simulink model "ECUDamperRR"  (Simulink 7.7)
settings: Solver=ode3  StartTime=0.0  StopTime=10.0  FixedStep=T  RelTol=1e-3
values from neighbouring files (symbols this model uses):
  Suspension =     [VehicleData_VectorCar.mat]
libraries: canoelib x5
settings Model: Creator=vishc  LastModifiedBy=visjf
settings DataIOCC: SaveOutput=off  SignalLogging=off  SaveTime=off
settings OptimizationCC: InlineParams=on  UseIntDivNetSlope=on
settings DebuggingCC: StrictBusMsg=Warning
settings SFSimCC: SimParseCustomCode=off
settings RTWCC: SystemTargetFile=cn.tlc  TemplateMakefile=cn_msdll.tmf  Description=Vector CANoe Real-Time Target DLL (Visual C/C++ Project Makefile)  ProcessScript=cn_make_rtw_hook
settings CodeAppCC: MaxIdLength=128  SimulinkBlockComments=off
settings STFCustomTargetCC: FunctionExecutionProfile=off  GeneratePreprocessorConditionals=Disable all  MatFileLogging=on  SystemTargetFile=cn.tlc
settings GRTTargetCC: ParMdlRefBuildCompliant=off  CompOptLevelCompliant=off  ExtModeMexFile=noextcomm  RTWCAPISignals=on  RTWCAPIParams=on
settings CustomProperty: DataType=string  Value=..\canoe

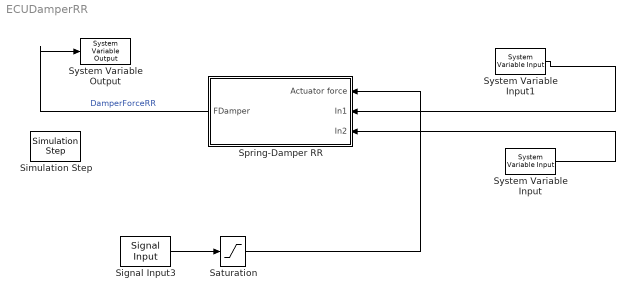
== system ECUDamperRR ==
  Saturation : Saturate  UpperLimit=6e3  LowerLimit=-6e3
  Signal Input3 : canoelib/CANoe I//O/Signal Input  SystemSampleTime=-1  dbName=""  nodeName=""  msgName=""  sigName=Susp_Ctrl_DesiredForce_RR  editSampleTime=0  rawValue=off
      settings: AttributesFormatString=%<sigName>
  Simulation Step : canoelib/CANoe I//O/Simulation Step  SystemSampleTime=-1  mode=Synchronized
      settings: AttributesFormatString=%<mode>
  Spring-Damper RR : Subsystem  AncestorBlock=vehicle_dynamics_lib/Force elements/Spring-Damper  mask{dtype=Active, pdamp=on, c=Suspension.SpringStiffnessLookUpRR, l0=Suspension.SpringFreeLengthRR, d=Suspension.DamperCushioningLookUpRR, d_s_max=1000}
      mask prompts: dtype "Damper type"; pdamp "With passive damper?"; c "Spring stiffness table [displacement ...;force ...]"; l0 "Spring free length [m]"; d "Damper cushioning table [velocity ...;force ...]"; d_s_max "Maximum active damper damping value [Ns/m]"
      settings: MinAlgLoopOccurrences=on
      mask StyleString: popup(Semi-active|Active|Passive),checkbox,edit,edit,edit,edit
      mask CallbackString:
      | % set control visibilities
      | pdamp = get_param(gcb,'pdamp');
      | if strcmpi(get_param(gcb,'dtype'),'active')
      |     set_param(gcb,'MaskVisibilities',{'on','on','on','on',pdamp,'off'});
      |     set_param(gcb,'pdamp',pdamp);
      | elseif strcmpi(get_param(gcb,'dtype'),'passive')
      |     set_param(gcb,'MaskVisibilities',{'on','off','on','on','on','off'});
      |     set_param(gcb,'pdamp','on');
      | else
      |     set_param(gcb,'MaskVisibilities',{'on','off','on','on','off','on'});
      |     set_param(gcb,'pdamp','off');
      | end
      | |tempvis = get_param(gcb,'MaskVisibilities');
      | if strcmpi(get_param(gcb,'pdamp'),'on')
      |     tempvis{5} = 'on';
      |     set_param(gcb,'MaskVisibilities',tempvis);
      | else
      |     tempvis{5} = 'off';
      |     set_param(gcb,'MaskVisibilities',tempvis);
      | end||||
      mask Display:
      | image(imread('damper.jpg'))
      | color('white')
      | port_label('input',2,'Actuator Force')
  System Variable Input : canoelib/CANoe I//O/System Variable Input  SystemSampleTime=-1  nsName=ModelDamper  sysVarName=Damper_RR1dot_suspvelocity  arrayIndex=-1  editSampleTime=0
      settings: AttributesFormatString=%<nsName>::%<sysVarName>
  System Variable Input1 : canoelib/CANoe I//O/System Variable Input  SystemSampleTime=-1  nsName=ModelDamper  sysVarName=Damper_RR_suspdeflection  arrayIndex=-1  editSampleTime=0
      settings: AttributesFormatString=%<nsName>::%<sysVarName>
  System Variable Output : canoelib/CANoe I//O/System Variable Output  SystemSampleTime=-1  nsName=ModelDamperForces  sysVarName=DamperForceRR  arrayIndex=-1
      settings: AttributesFormatString=%<nsName>::%<sysVarName>
  wires:
  Spring-Damper RR/1(FDamper) -> System Variable Output/1  "DamperForceRR"
  Signal Input3/1 -> Saturation/1
  Saturation/1 -> Spring-Damper RR/1(Actuator force)
  System Variable Input1/1 -> Spring-Damper RR/2(In1)
  System Variable Input/1 -> Spring-Damper RR/3(In2)

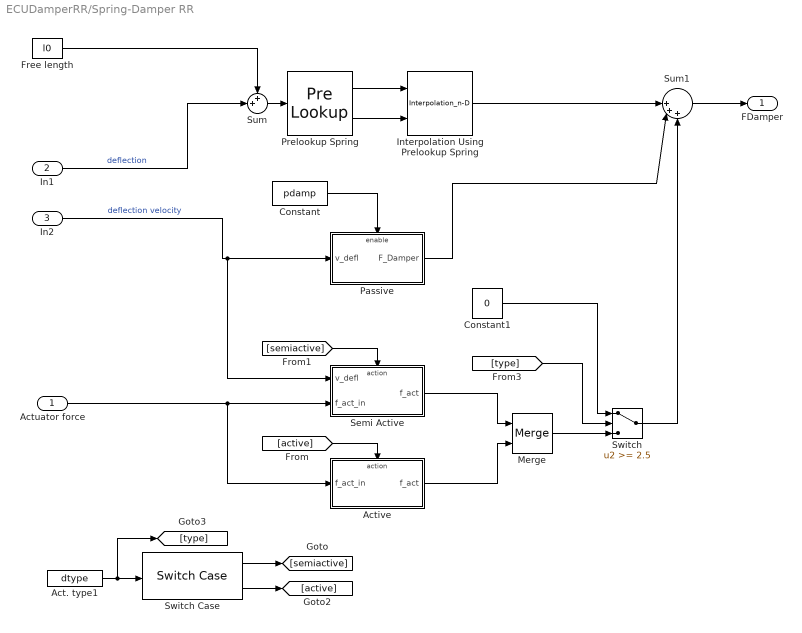
== system ECUDamperRR/Spring-Damper RR ==
  Actuator force : Inport
  In1 : Inport  Port=2
  In2 : Inport  Port=3
  Act. type1 : Constant  Value=dtype
      settings: AttributesFormatString=1 = semi-active\n2 = active\n3 = passive
  Active : Subsystem  TreatAsAtomicUnit=on
  Constant : Constant  Value=pdamp
  Constant1 : Constant  Value=0
  Free length : Constant  Value=l0
  Interpolation Using Prelookup Spring : Interpolation_n-D  NumberOfTableDimensions=1  Table=c(2,:)
      settings: InputPortMap=u0,u1
  Merge : Merge
  Passive : Subsystem  TreatAsAtomicUnit=on
  Prelookup Spring : PreLookup  BreakpointsData=c(1,:)  ExtrapMethod=Linear
  Semi Active : Subsystem  TreatAsAtomicUnit=on
  Sum : Sum  Inputs=++|
  Sum1 : Sum  Inputs=||+++
  Switch : Switch  Threshold=2.5
  Switch Case : SwitchCase  CaseConditions={1,2}  ShowDefaultCase=off
  FDamper : Outport
  wires:
  Merge/1 -> Switch/3
  Constant1/1 -> Switch/1
  Switch/1 -> Sum1/3
  Semi Active/1(f_act) -> Merge/1
  Active/1(f_act) -> Merge/2
  Passive/1(F_Damper) -> Sum1/2
  Constant/1 -> Passive/Enable
  [type] -> Switch/2
  [semiactive] -> Semi Active/Action
  [active] -> Active/Action
  Switch Case/2 -> [active]
  Switch Case/1 -> [semiactive]
  Actuator force/1 -> Active/1(f_act_in), Semi Active/2(f_act_in)
  Act. type1/1 -> [type], Switch Case/1
  Prelookup Spring/1 -> Interpolation Using Prelookup Spring/1
  Prelookup Spring/2 -> Interpolation Using Prelookup Spring/2
  Sum/1 -> Prelookup Spring/1
  Free length/1 -> Sum/1
  Sum1/1 -> FDamper/1
  Interpolation Using Prelookup Spring/1 -> Sum1/1
  In1/1 -> Sum/2  "deflection"
  In2/1 -> Semi Active/1(v_defl), Passive/1(v_defl)  "deflection velocity"

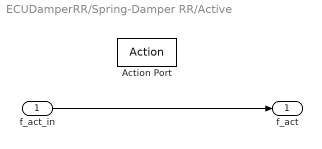
== system ECUDamperRR/Spring-Damper RR/Active ==
  f_act_in : Inport
  Action Port : ActionPort  ActionType=case
  f_act : Outport
  wires:
  f_act_in/1 -> f_act/1

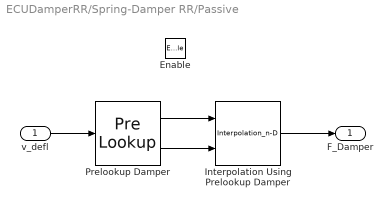
== system ECUDamperRR/Spring-Damper RR/Passive ==
  v_defl : Inport
  Enable : EnablePort  StatesWhenEnabling=reset
  Interpolation Using Prelookup Damper : Interpolation_n-D  NumberOfTableDimensions=1  Table=d(2,:)
      settings: InputPortMap=u0,u1
  Prelookup Damper : PreLookup  BreakpointsData=d(1,:)  ExtrapMethod=Linear
  F_Damper : Outport  OutputWhenDisabled=reset  InitialOutput=0
  wires:
  Interpolation Using Prelookup Damper/1 -> F_Damper/1
  v_defl/1 -> Prelookup Damper/1
  Prelookup Damper/1 -> Interpolation Using Prelookup Damper/1
  Prelookup Damper/2 -> Interpolation Using Prelookup Damper/2

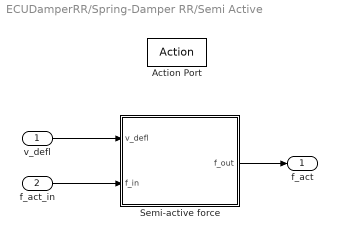
== system ECUDamperRR/Spring-Damper RR/Semi Active ==
  v_defl : Inport
  f_act_in : Inport  Port=2
  Action Port : ActionPort  ActionType=case
  Semi-active force : Stateflow chart  TreatAsAtomicUnit=on
  f_act : Outport
  wires:
  v_defl/1 -> Semi-active force/1(v_defl)
  f_act_in/1 -> Semi-active force/2(f_in)
  Semi-active force/1(f_out) -> f_act/1

== matlab function Spring-Damper RR/Semi Active/Semi-active force ==
  data: v_defl input double size=1; f_out output double size=1; f_in input double size=1; d_s_max parameter double
function f_out = semiact(v_defl,f_in,d_s_max)
%#eml

if( f_in * v_defl > 0 )
    f_out = sign(f_in)*min(d_s_max*abs(v_defl),abs(f_in));
else
    f_out = 0;
end
